simulink model "doc_punct"  (R2014a)
settings: Solver=VariableStepDiscrete  SolverMode=SingleTasking  StartTime=0.0  StopTime=inf  RelTol=1e-3
values from neighbouring files (symbols this model uses):
  delay = N/(nSamp*2)    (= 5)    [commdoc_code.m]
undefined symbols (not defined in the file or in its folder): commblksprivate, Info
libraries: commcnvcod2 x2, commsink2 x2, commdigbbndpm3 x2, commfilt2 x2, commutil2 x1, commchan3 x1, commrandsrc2 x1, dspsigops x1
settings Model: RequirementInfo=9  CovMetricSettings=d  ExtModeTrigMode=oneshot  ExtModeArmWhenConnect=off  ExtModeAutoUpdateStatusClock=off  Creator=The MathWorks Inc.
settings DataIOCC: LimitDataPoints=off  SignalLoggingSaveFormat=ModelDataLogs  SaveOutput=off  SaveTime=off  SignalLoggingName=sigsOut
settings OptimizationCC: BlockReduction=off  BooleanDataType=off  ExpressionDepthLimit=2147483647  InitFltsAndDblsToZero=on
settings DebuggingCC: SaveWithParameterizedLinksMsg=none  UnderspecifiedInitializationDetection=Classic  CheckExecutionContextPreStartOutputMsg=on  CheckExecutionContextRuntimeOutputMsg=on  SignalResolutionControl=TryResolveAllWithWarning  SolverPrmCheckMsg=none  InheritedTsInSrcMsg=none  MultiTaskDSMMsg=warning  MultiTaskCondExecSysMsg=none  SigSpecEnsureSampleTimeMsg=none  IntegerOverflowMsg=none  FcnCallInpInsideContextMsg=UseLocalSettings  StateNameClashWarn=warning
settings HardwareCC: TargetUnknown=on
settings ModelReferenceCC: UpdateModelReferenceTargets=IfOutOfDate
settings RTWCC: IncludeERTFirstTime=on
settings GRTTargetCC: TargetFcnLib=ansi_tfl_tmw.mat  CombineOutputUpdateFcns=off  GRTInterface=on

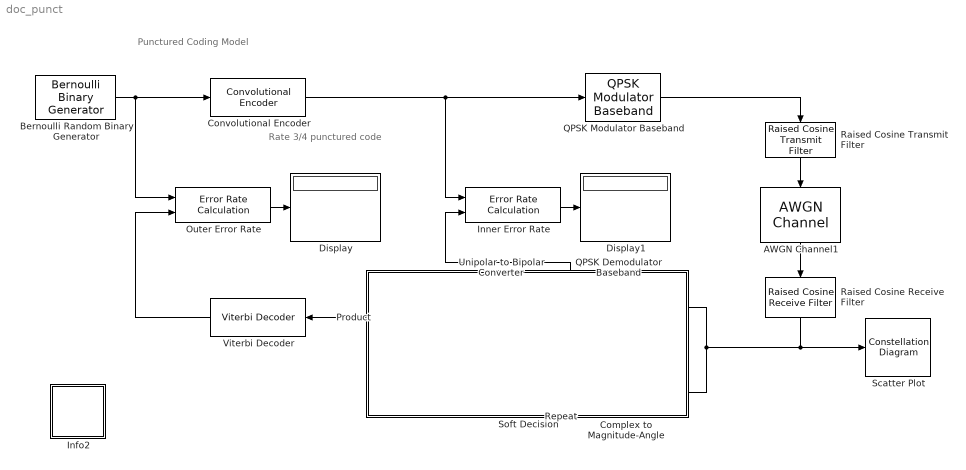
== system doc_punct ==
  note: Rate 3/4 punctured code
  note: Punctured Coding Model
  " Unipolar to Bipolar Converter" : commutil2/Unipolar to Bipolar Converter  M=2  polarity=Negative  dataType=Inherit via internal rule
  AWGN Channel1 : commchan3/AWGN Channel  InputProcessing=Columns as channels (frame based)  seed=123456  noiseMode="Signal to noise ratio  (Es/No)"  EbNodB=10  EsNodB=7  SNRdB=10  bitsPerSym=1  Ps=1/8  Tsym=3/2*5.5e-5  variance=1
  Bernoulli Random Binary Generator : commrandsrc2/Bernoulli Binary Generator  P=0.5  seed=101  Ts=5.5e-5  frameBased=on  sampPerFrame=3  orient=off  outDataType=double
  Complex to Magnitude-Angle : ComplexToMagnitudeAngle  Output=Magnitude
  Convolutional Encoder : commcnvcod2/Convolutional Encoder  trellis=poly2trellis(7, [171 133])  opMode=Continuous  DelayedResetAction=off  hasIniStPort=off  hasFinStPort=off  usePuncVector=on  punctureVector=[1 1 0 1 1 0].'  reset=Unused parameter value
  Display : Display
  Display1 : Display
  Info2 : Subsystem  AncestorBlock=commblksprivate/Info  mask(Info){}
      settings: OpenFcn=helpview([docroot '/toolbox/comm/comm.map'], 'doc_punct');
      mask Display: disp('Info')
  Inner Error Rate : commsink2/Error Rate Calculation  N="(2 + 3 + 3) * 2  % (Initial frame delay + Tx filter delay + Rx filter delay) * (2 bits per QPSK symbol)"  st_delay=0  cp_mode=Entire frame  subframe=[]  PMode=Port  WsName=ErrorVec  RsMode2=off  stop=off  numErr=300  maxBits=1e6
  Outer Error Rate : commsink2/Error Rate Calculation  N=(3/2+3/2+1)*3+96  st_delay=0  cp_mode=Entire frame  subframe=[]  PMode=Port  WsName=ErrorVec  RsMode2=off  stop=on  numErr=50  maxBits=1e6
  Product : Product  SaturateOnIntegerOverflow=on  InputSameDT=on  OutDataTypeStr=Inherit: Same as first input
  QPSK Demodulator Baseband : commdigbbndpm3/QPSK Demodulator Baseband  Ph=pi/4  Dec=Gray  OutType=Bit  DecType=Hard decision  VarSource=Dialog  Variance=1  outDtype1=double  outDtype2=double  derotateFactorWordLen=16
  QPSK Modulator Baseband : commdigbbndpm3/QPSK Modulator Baseband  InType=Bit  Enc=Gray  Ph=pi/4  outDtype=double  outWordLen=16  outUDDataType=sfix(16)  outFracLenMode=Best precision  outFracLen=15
  Raised Cosine Receive Filter : commfilt2/Raised Cosine Receive Filter  filtType=Square root  N=8  filtSpan=6  currentFiltSpan=6  D=(6)/2  R=0.5  sampMode=Mute  saveAsFlag=0  rateMode=Downsampling  downFactor=8  downOffset=0  framing=Allow multirate processing  InputProcessing=Columns as channels (frame based)  checkGain=Normalized  filterGain=1  checkCoeff=off  variableName=rcRxFilt  launchFVT=off  roundingMode=Floor  overflowMode=off
  Raised Cosine Transmit Filter : commfilt2/Raised Cosine Transmit Filter  filtType=Square root  filtSpan=6  currentFiltSpan=6  D=(6)/2  R=0.5  sampMode=Mute  saveAsFlag=0  N=8  framing=Allow multirate processing  InputProcessing=Columns as channels (frame based)  checkGain=Normalized  filterGain=1  checkCoeff=off  variableName=rcTxFilt  launchFVT=off  roundingMode=Floor  overflowMode=off
  Repeat : dspsigops/Repeat  N=2  InputProcessing=Inherited (this choice will be removed - see release notes)  RateOptions=Enforce single-rate processing  ic=0  mode=Unused parameter value
  Scatter Plot : ConstellationDiagram  Tag=ScatterPlot
  Soft Decision : Subsystem
      mask Display: disp('')
  Viterbi Decoder : commcnvcod2/Viterbi Decoder  trellis=poly2trellis(7, [171 133])  isPunctured=on  punctureVector=[1 1 0 1 1 0].'  erasures=off  dectype=Unquantized  runSigValErrCheck=off  nsdecb=4  smWordLength=16  tbdepth=96  opmode=Continuous  reset=off  outDataType=double  delayedResetAction=off
  wires:
  QPSK Modulator Baseband/1 -> Raised Cosine Transmit Filter/1
  Complex to Magnitude-Angle/1 -> Repeat/1
  Outer Error Rate/1 -> Display/1
  Inner Error Rate/1 -> Display1/1
  Product/1 -> Viterbi Decoder/1
  " Unipolar to Bipolar Converter"/1 -> Product/1
  Repeat/1 -> Product/2
  Bernoulli Random Binary Generator/1 -> Convolutional Encoder/1, Outer Error Rate/1
  Viterbi Decoder/1 -> Outer Error Rate/2
  Raised Cosine Transmit Filter/1 -> AWGN Channel1/1
  AWGN Channel1/1 -> Raised Cosine Receive Filter/1
  Raised Cosine Receive Filter/1 -> Scatter Plot/1, Complex to Magnitude-Angle/1, QPSK Demodulator Baseband/1
  QPSK Demodulator Baseband/1 -> Inner Error Rate/2, " Unipolar to Bipolar Converter"/1
  Convolutional Encoder/1 -> QPSK Modulator Baseband/1, Inner Error Rate/1

== system doc_punct/Info2 ==

== system doc_punct/Soft Decision ==
